simulink library "BlockLib"  (R2014b)
settings: Solver=ode45  StartTime=0.0  StopTime=10.0  RelTol=1e-3
undefined symbols (not defined in the file or in its folder): beamSplitterReflect, beamSplitterTransmit, delay, halfWavePlate, linearPolarizer, pockelsCell, polBeamSplitterReflect, polBeamSplitterTransmit, signalSampler
libraries: BlockLib x3
settings Model: Creator=kunalmenda  LastModifiedBy=kunalmenda

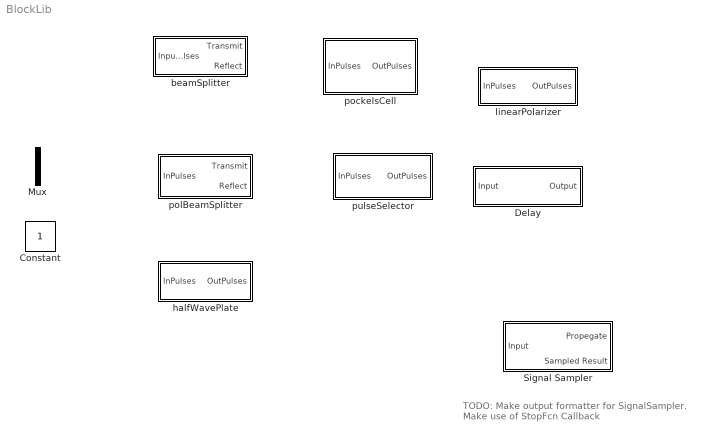
== system BlockLib ==
  note: TODO: Make output formatter for SignalSampler.
      |  Make use of StopFcn Callback
  Constant : Constant
  Delay : Subsystem  mask{DelayAmt=1}
      mask TypeOptions DelayAmt: DelayAmt/Value
  Mux : Mux  Inputs=2
  Signal Sampler : Subsystem
  "beamSplitter " : Subsystem
  halfWavePlate : Subsystem  mask{AxisAngle=1}
      mask TypeOptions AxisAngle: AxisAngle/Value
  linearPolarizer : Subsystem  mask{AxisAngle=1}
      mask TypeOptions AxisAngle: AxisAngle/Value
  pockelsCell : Subsystem  mask{OutputDimensions=-1, AxisAngle=1, PCID=-1}
      mask prompts: OutputDimensions "Simulink:blkprm_prompts:MATLABFcnOutDims"; AxisAngle "Axis Angle:"
      mask TypeOptions OutputDimensions:
      | Interpreted MATLAB
      | Function/OutputDimensions
      mask TypeOptions AxisAngle: AxisAngle/Value
      mask TypeOptions PCID: PCID/Value
  polBeamSplitter : Subsystem
  pulseSelector : Subsystem  mask{OutputDimensions=-1, PCID=-1}
      mask prompts: OutputDimensions "Output Dimensions"
      mask TypeOptions OutputDimensions: pockelsCell/OutputDimensions
      mask TypeOptions PCID: pockelsCell/PCID

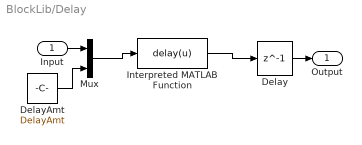
== system BlockLib/Delay ==
  Input : Inport
  Delay : Delay  DelayLength=1  InitialCondition=0
  DelayAmt : Constant  Value=DelayAmt
  Interpreted MATLAB Function : MATLABFcn  MATLABFcn=delay(u)
  Mux : Mux  Inputs=2
  Output : Outport
  wires:
  Mux/1 -> Interpreted MATLAB Function/1
  Delay/1 -> Output/1
  Input/1 -> Mux/1
  Interpreted MATLAB Function/1 -> Delay/1
  DelayAmt/1 -> Mux/2

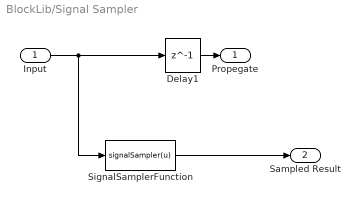
== system BlockLib/Signal Sampler ==
  Input : Inport
  Delay1 : Delay  DelayLength=1  InitialCondition=0
  SignalSamplerFunction : MATLABFcn  MATLABFcn=signalSampler(u)
  Propegate : Outport
  Sampled Result : Outport  Port=2
  wires:
  SignalSamplerFunction/1 -> Sampled Result/1
  Delay1/1 -> Propegate/1
  Input/1 -> SignalSamplerFunction/1, Delay1/1

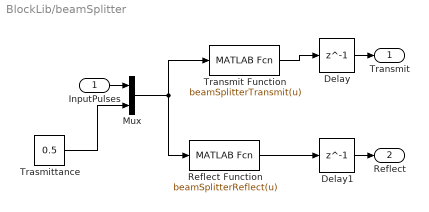
== system BlockLib/beamSplitter  ==
  InputPulses : Inport
  Delay : Delay  DelayLength=1  InitialCondition=0
  Delay1 : Delay  DelayLength=1  InitialCondition=0
  Mux : Mux  Inputs=2
  Reflect Function : MATLABFcn  MATLABFcn=beamSplitterReflect(u)
  Transmit Function : MATLABFcn  MATLABFcn=beamSplitterTransmit(u)
  Trasmittance : Constant  Value=0.5
  Transmit : Outport
  Reflect : Outport  Port=2
  wires:
  Mux/1 -> Transmit Function/1, Reflect Function/1
  Delay1/1 -> Reflect/1
  Delay/1 -> Transmit/1
  InputPulses/1 -> Mux/1
  Trasmittance/1 -> Mux/2
  Transmit Function/1 -> Delay/1
  Reflect Function/1 -> Delay1/1

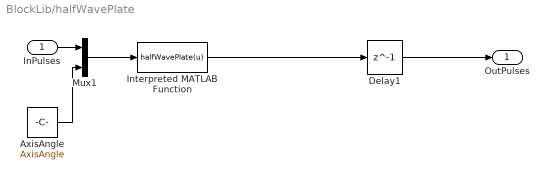
== system BlockLib/halfWavePlate ==
  InPulses : Inport
  AxisAngle : Constant  Value=AxisAngle
  Delay1 : Delay  DelayLength=1  InitialCondition=0
  Interpreted MATLAB Function : MATLABFcn  MATLABFcn=halfWavePlate(u)
  Mux1 : Mux  Inputs=2
  OutPulses : Outport
  wires:
  InPulses/1 -> Mux1/1
  Delay1/1 -> OutPulses/1
  Mux1/1 -> Interpreted MATLAB Function/1
  AxisAngle/1 -> Mux1/2
  Interpreted MATLAB Function/1 -> Delay1/1

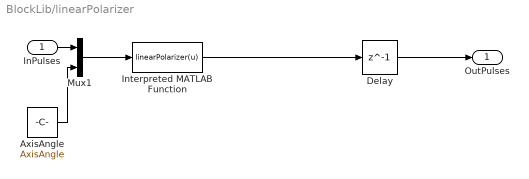
== system BlockLib/linearPolarizer ==
  InPulses : Inport
  AxisAngle : Constant  Value=AxisAngle
  Delay : Delay  DelayLength=1  InitialCondition=0
  Interpreted MATLAB Function : MATLABFcn  MATLABFcn=linearPolarizer(u)
  Mux1 : Mux  Inputs=2
  OutPulses : Outport
  wires:
  AxisAngle/1 -> Mux1/2
  InPulses/1 -> Mux1/1
  Mux1/1 -> Interpreted MATLAB Function/1
  Interpreted MATLAB Function/1 -> Delay/1
  Delay/1 -> OutPulses/1

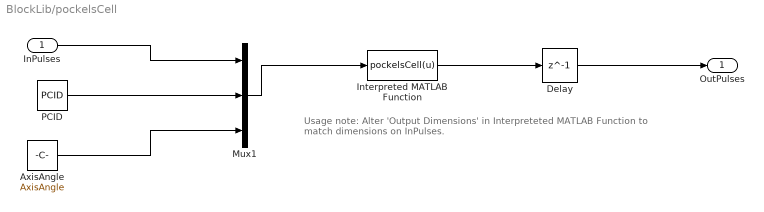
== system BlockLib/pockelsCell ==
  note: Usage note: Alter 'Output Dimensions' in Interpreteted MATLAB Function
      |  to match dimensions on InPulses.
  InPulses : Inport
  AxisAngle : Constant  Value=AxisAngle
  Delay : Delay  DelayLength=1  InitialCondition=0
  Interpreted MATLAB Function : MATLABFcn  MATLABFcn=pockelsCell(u)  OutputDimensions=OutputDimensions
  Mux1 : Mux  Inputs=3
  PCID : Constant  Value=PCID
  OutPulses : Outport
  wires:
  Mux1/1 -> Interpreted MATLAB Function/1
  InPulses/1 -> Mux1/1
  Interpreted MATLAB Function/1 -> Delay/1
  Delay/1 -> OutPulses/1
  AxisAngle/1 -> Mux1/3
  PCID/1 -> Mux1/2

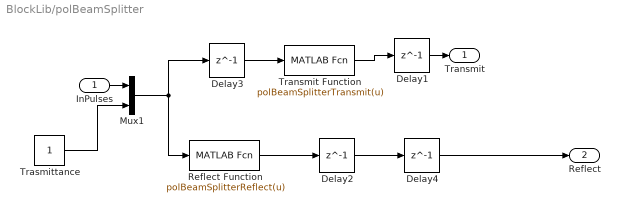
== system BlockLib/polBeamSplitter ==
  InPulses : Inport
  Delay{1..4} (4 alike) : Delay  DelayLength=1  InitialCondition=0
  Mux1 : Mux  Inputs=2
  Reflect Function : MATLABFcn  MATLABFcn=polBeamSplitterReflect(u)
  Transmit Function : MATLABFcn  MATLABFcn=polBeamSplitterTransmit(u)
  Trasmittance : Constant
  Transmit : Outport
  Reflect : Outport  Port=2
  wires:
  Trasmittance/1 -> Mux1/2
  Transmit Function/1 -> Delay1/1
  InPulses/1 -> Mux1/1
  Delay1/1 -> Transmit/1
  Mux1/1 -> Reflect Function/1, Delay3/1
  Reflect Function/1 -> Delay2/1
  Delay3/1 -> Transmit Function/1
  Delay2/1 -> Delay4/1
  Delay4/1 -> Reflect/1

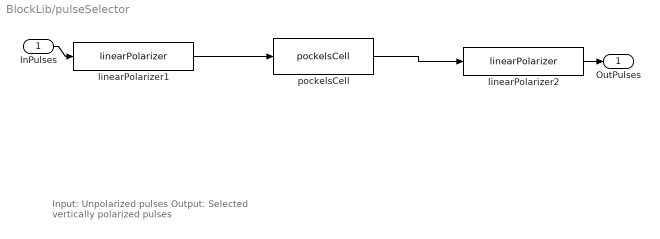
== system BlockLib/pulseSelector ==
  note: Input: Unpolarized pulses
      | Output: Selected vertically polarized pulses
  InPulses : Inport
  linearPolarizer1 : BlockLib/linearPolarizer  AxisAngle=0
  linearPolarizer2 : BlockLib/linearPolarizer  AxisAngle=pi/2
  pockelsCell : BlockLib/pockelsCell  OutputDimensions=OutputDimensions  AxisAngle=pi/4  PCID=PCID
  OutPulses : Outport
  wires:
  linearPolarizer2/1 -> OutPulses/1
  InPulses/1 -> linearPolarizer1/1
  linearPolarizer1/1 -> pockelsCell/1
  pockelsCell/1 -> linearPolarizer2/1
